simulink model "real world"  (R2020b)
settings: Solver=VariableStepAuto  StartTime=0.0  StopTime=10.0  RelTol=1e-3
settings Model: Creator=99003184  LastModifiedBy=99003178

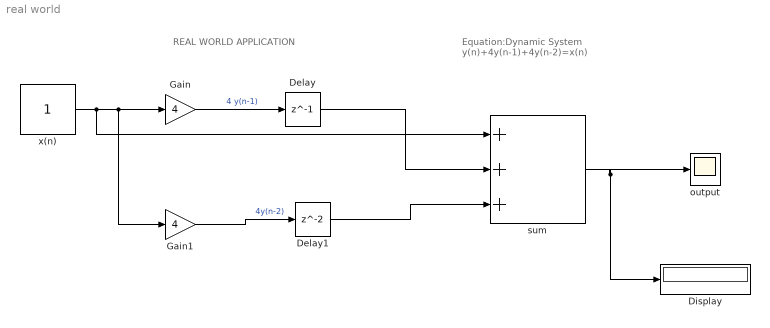
== system real world ==
  note: Equation:Dynamic System
      | y(n)+4y(n-1)+4y(n-2)=x(n)
  note: REAL WORLD APPLICATION
  Delay : Delay  DelayLength=1
  Delay1 : Delay
  Display : Display
  Gain : Gain  Gain=4
  Gain1 : Gain  Gain=4
  output : Scope
  sum : Sum  Inputs=+++
  x(n) : Constant
  wires:
  x(n)/1 -> sum/1, Gain1/1, Gain/1
  Gain/1 -> Delay/1  "4 y(n-1)"
  Delay/1 -> sum/2
  Gain1/1 -> Delay1/1  "4y(n-2)"
  Delay1/1 -> sum/3
  sum/1 -> Display/1, output/1
